simulink model "StSys_AddCor"  (R2016b)
settings: configuration reference "CodeGenConfigSet" (kept outside this file)
values from neighbouring files (symbols this model uses):
  StSys_facStrtAPS_CUR = Calibration.Parameter    [init_StSys_AddCor.m]    (also in init_StSys_AddCor_SIL.m = Simulink.Parameter)
  StSys_facStrtAPS_CURX = Calibration.Parameter    [init_StSys_AddCor.m]    (also in init_StSys_AddCor_SIL.m = Simulink.Parameter)
  StSys_trqStrtAPS_MAP = Calibration.Parameter    [init_StSys_AddCor.m]    (also in init_StSys_AddCor_SIL.m = Simulink.Parameter)
  StSys_trqStrtAPS_MAPX = Calibration.Parameter    [init_StSys_AddCor.m]    (also in init_StSys_AddCor_SIL.m = Simulink.Parameter)
  StSys_trqStrtAPS_MAPY = Calibration.Parameter    [init_StSys_AddCor.m]    (also in init_StSys_AddCor_SIL.m = Simulink.Parameter)
settings Model: Creator=Colin  LastModifiedBy=zhoutinglin
settings ConfigSetRef: SourceLocation=Base Workspace

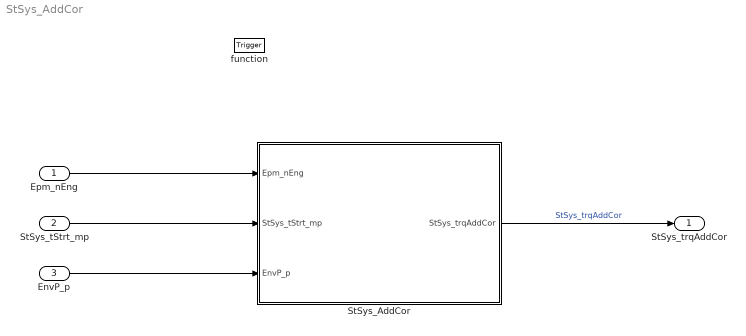
== system StSys_AddCor ==
  Epm_nEng : Inport  Tag=rpm  Description=Engine speed  OutMin=0  OutMax=6000  OutDataTypeStr=EngSpeed_rpm
  StSys_tStrt_mp : Inport  Tag=deg  Description=engine temperature for starting system  Port=2  OutMin=-50  OutMax=150  OutDataTypeStr=Temp_deg
  EnvP_p : Inport  Tag=kPa  Description=Barometric pressure  Port=3  OutMin=0  OutMax=3276  OutDataTypeStr=AirPressure_kPa
  function : TriggerPort  TriggerType=function-call  VariantControl=Variant
  StSys_AddCor : Subsystem
  StSys_trqAddCor : Outport  Tag=Nm  Description=additional correction torque for starting torque  OutMin=-1000  OutMax=1000  OutDataTypeStr=Trq_Nm
  wires:
  StSys_AddCor/1(StSys_trqAddCor) -> StSys_trqAddCor/1  "StSys_trqAddCor"
  Epm_nEng/1 -> StSys_AddCor/1(Epm_nEng)
  StSys_tStrt_mp/1 -> StSys_AddCor/2(StSys_tStrt_mp)
  EnvP_p/1 -> StSys_AddCor/3(EnvP_p)

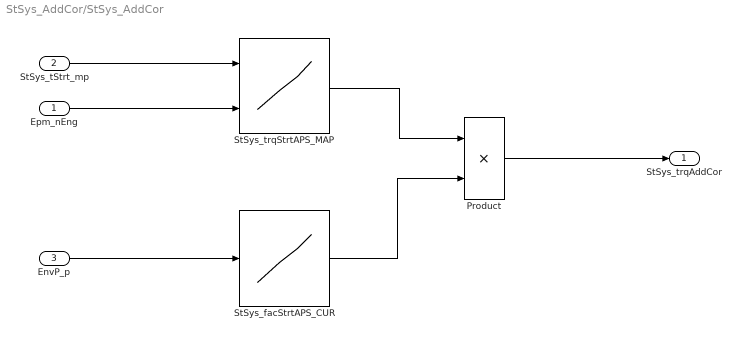
== system StSys_AddCor/StSys_AddCor ==
  Epm_nEng : Inport  Tag=rpm  Description=Engine Speed  OutMin=0  OutMax=6000  OutDataTypeStr=EngSpeed_rpm
  StSys_tStrt_mp : Inport  Tag=deg  Description=engine temperature for starting system  Port=2  OutMin=-50  OutMax=150  OutDataTypeStr=Temp_deg
  EnvP_p : Inport  Tag=kPa  Description=Barometric pressure  Port=3  OutMin=0  OutMax=300  OutDataTypeStr=AirPressure_kPa
  Product : Product  OutDataTypeStr=Inherit: Inherit via back propagation  SaturateOnIntegerOverflow=on
  StSys_facStrtAPS_CUR : Lookup_n-D  NumberOfTableDimensions=1  BreakpointsForDimension1=StSys_facStrtAPS_CURX  Table=StSys_facStrtAPS_CUR  TableDataTypeStr=Inherit: Inherit from 'Table data'  ExtrapMethod=Clip  InternalRulePriority=Speed  OutDataTypeStr=Inherit: Inherit from 'Table data'  RndMeth=Simplest  InputSameDT=on
  StSys_trqStrtAPS_MAP : Lookup_n-D  BreakpointsForDimension1=StSys_trqStrtAPS_MAPY  BreakpointsForDimension2=StSys_trqStrtAPS_MAPX  BreakpointsForDimension1DataTypeStr=Inherit: Inherit from 'Breakpoint data'  BreakpointsForDimension2DataTypeStr=Inherit: Inherit from 'Breakpoint data'  Table=StSys_trqStrtAPS_MAP  TableDataTypeStr=Inherit: Inherit from 'Table data'  ExtrapMethod=Clip  InternalRulePriority=Speed  OutDataTypeStr=Inherit: Inherit from 'Table data'  RndMeth=Simplest
  StSys_trqAddCor : Outport  Tag=Nm  Description=additional correction torque for starting torque  OutMin=0  OutMax=1000  OutDataTypeStr=Trq_Nm
  wires:
  EnvP_p/1 -> StSys_facStrtAPS_CUR/1
  StSys_tStrt_mp/1 -> StSys_trqStrtAPS_MAP/1
  Epm_nEng/1 -> StSys_trqStrtAPS_MAP/2
  StSys_trqStrtAPS_MAP/1 -> Product/1
  StSys_facStrtAPS_CUR/1 -> Product/2
  Product/1 -> StSys_trqAddCor/1
